simulink model "V5_2016_1"  (R2016a)
settings: Solver=VariableStepAuto  SolverMode=SingleTasking  StartTime=0.0  StopTime=60  RelTol=1e-3
values from neighbouring files (symbols this model uses):
  Ar = pi * (Lr^2) / 4    (= 0.0126676869774)    [Barrowman_Equations.m]    (also in barrowaman.mat)
  CD_data = CD{:, 2}    [Barrowman_Equations.m]    (also in barrowaman.mat = [0.48 0.48 0.47 0.46 0.45 0.44 0.43 0.42 0.42 0.41 0.4 0.4 .)
  CD_input = CD{:, 1}    [Barrowman_Equations.m]    (also in barrowaman.mat = [0.01 0.02 0.03 0.04 0.05 0.06 0.07 0.08 0.09 0.1 0.11 0.12 )
  Cnalfa = (Cnab + Cnalfat + Cntail)    [Barrowman_Equations.m]    (also in barrowaman.mat = 8.08141723415)
  Cndomega = (N * Cnalfa0 * Lr * (c1 + c2 + c3))/(Ar * span * (Lr))    [Barrowman_Equations.m]
  Cnfdelta = N * Cnalfa1 * Y / span    [Barrowman_Equations.m]    (also in barrowaman.mat = 4.20666666667)
  delta = pi/60    (= 0.0523598775598)    [Barrowman_Equations.m]    (also in barrowaman.mat = 0.00872664625997)
  F = readtable('Data/Comercial/Pro75M3100_saida_do_trilho.csv')    [Barrowman_Equations.m]
  F_data = F{:, 2}    [Barrowman_Equations.m]    (also in barrowaman.mat = [3391.768 3665.504 3532.913 3357.551 3199.297 3139.417 2412.)
  F_input = F{:, 1}    [Barrowman_Equations.m]    (also in barrowaman.mat = [0.02 0.057 0.148 0.496 0.817 0.936 1.173 1.501 1.717 1.78 1)
  mdescarregado = 15.576    [Barrowman_Equations.m]    (also in barrowaman.mat)
  MDot_data = MDot{:, 2}    [Barrowman_Equations.m]    (also in barrowaman.mat = [-1.96086837808 -2.11912220509 -2.04246793537 -1.9410866497 )
  MDot_input = MDot{:, 1}    [Barrowman_Equations.m]    (also in barrowaman.mat = [0.02 0.057 0.148 0.496 0.817 0.936 1.173 1.501 1.717 1.78 1)
  r = rt/r2    (= 1.45977011494)    [Barrowman_Equations.m]    (also in barrowaman.mat)
  x_cg = -1.278    [Barrowman_Equations.m]    (also in barrowaman.mat)
  x_ref = (XB * Cnab + XTB * Cnalfat + Xtail * Cntail) / Cnalfa    [Barrowman_Equations.m]    (also in barrowaman.mat = -1.69759908608)
undefined symbols (not defined in the file or in its folder): Light, MIL
libraries: aerolibasang x3, aerolibwind2 x3, aerolibatmos2 x1, aerolib6dof2 x1
settings Model: Creator=bruno  LastModifiedBy=patri
settings DataIOCC: ReturnWorkspaceOutputs=on
settings DebuggingCC: SFUnexpectedBacktrackingDiag=error  SFNoUnconditionalDefaultTransitionDiag=error
settings SFSimCC: SimUseLocalCustomCode=on
settings RTWCC: RTWUseLocalCustomCode=on
settings GRTTargetCC: TargetLangStandard=C99 (ISO)  GeneratePreprocessorConditionals=Use local settings
settings ConfigComp: CovMetricSettings=dwe  CovHtmlReporting=off  CovSaveCumulativeToWorkspaceVar=off  CovSaveSingleToWorkspaceVar=off  CovExternalEMLEnable=on

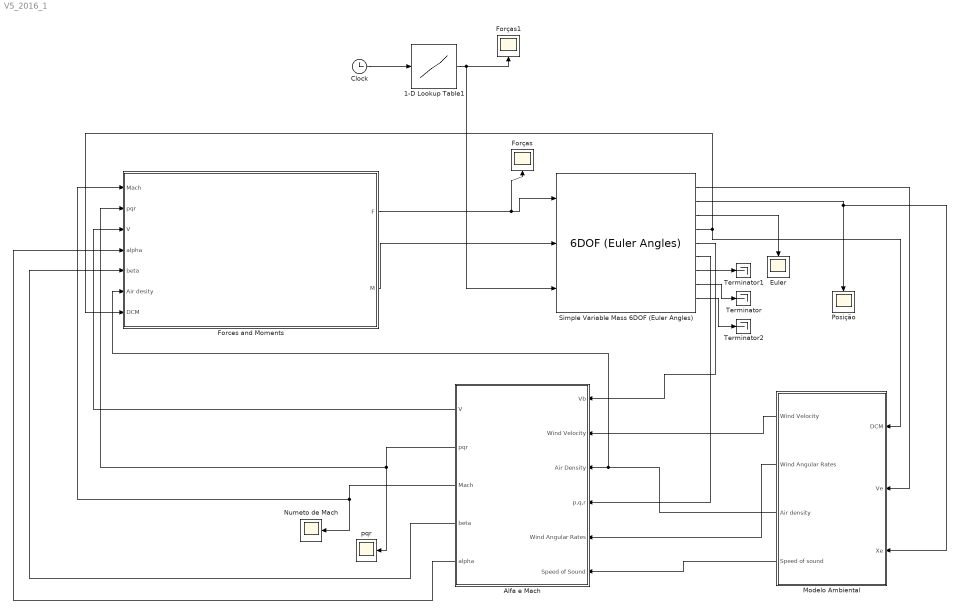
== system V5_2016_1 ==
  1-D Lookup Table1 : Lookup_n-D  NumberOfTableDimensions=1  BreakpointsForDimension1=MDot_input  Table=MDot_data  InternalRulePriority=Speed  RndMeth=Simplest  InputSameDT=on
  Alfa e Mach : Subsystem
  Clock : Clock
  Euler : Scope
  "Forces and Moments " : Subsystem
  Forças : Scope
  Forças1 : Scope
  Modelo Ambiental : Subsystem
  Numeto de Mach : Scope
  "Posição " : Scope
  Simple Variable Mass 6DOF (Euler Angles) : aerolib6dof2/6DOF (Euler Angles)  units=Metric (MKS)  mtype=Simple Variable  rep=Euler Angles  xme_0=[5 0 0]  Vm_0=[38 0 0]  eul_0=[0 -pi/2 0]  pm_0=[0 0 0]  mass_0=mcarregado  mass_e=mdescarregado  mass_f=mcarregado  inertia=eye(3)  inertia_e=MatrizDeInerciaDescarregado  inertia_f=MatrizDeInercia  k_quat=1.0  vre_flag=off
  Terminator : Terminator
  Terminator1 : Terminator
  Terminator2 : Terminator
  "pqr " : Scope
  wires:
  Simple Variable Mass 6DOF (Euler Angles)/4 -> Modelo Ambiental/1(DCM), "Forces and Moments "/7(DCM)
  Simple Variable Mass 6DOF (Euler Angles)/1 -> Modelo Ambiental/2(Ve)
  Simple Variable Mass 6DOF (Euler Angles)/2 -> "Posição "/1, Modelo Ambiental/3(Xe)
  Modelo Ambiental/3(Air density) -> "Forces and Moments "/6(Air desity), Alfa e Mach/3(Air Density)
  Modelo Ambiental/1(Wind Velocity) -> Alfa e Mach/2(Wind Velocity)
  Simple Variable Mass 6DOF (Euler Angles)/5 -> Alfa e Mach/1(Vb)
  Simple Variable Mass 6DOF (Euler Angles)/6 -> Alfa e Mach/4(p,q,r)
  Modelo Ambiental/4(Speed of sound) -> Alfa e Mach/6(Speed of Sound)
  Modelo Ambiental/2(Wind Angular Rates) -> Alfa e Mach/5(Wind Angular Rates)
  Alfa e Mach/3(Mach) -> Numeto de Mach/1, "Forces and Moments "/1(Mach)
  Alfa e Mach/2(pqr) -> "pqr "/1, "Forces and Moments "/2(pqr)
  Alfa e Mach/1(V) -> "Forces and Moments "/3("V ")
  Simple Variable Mass 6DOF (Euler Angles)/3 -> Euler/1
  Alfa e Mach/5("alpha ") -> "Forces and Moments "/4("alpha ")
  Alfa e Mach/4(beta) -> "Forces and Moments "/5(beta)
  "Forces and Moments "/1(F) -> Simple Variable Mass 6DOF (Euler Angles)/1, Forças/1
  Simple Variable Mass 6DOF (Euler Angles)/7 -> Terminator1/1
  Simple Variable Mass 6DOF (Euler Angles)/8 -> Terminator/1
  Clock/1 -> 1-D Lookup Table1/1
  1-D Lookup Table1/1 -> Simple Variable Mass 6DOF (Euler Angles)/3, Forças1/1
  Simple Variable Mass 6DOF (Euler Angles)/9 -> Terminator2/1
  "Forces and Moments "/2(M) -> Simple Variable Mass 6DOF (Euler Angles)/2

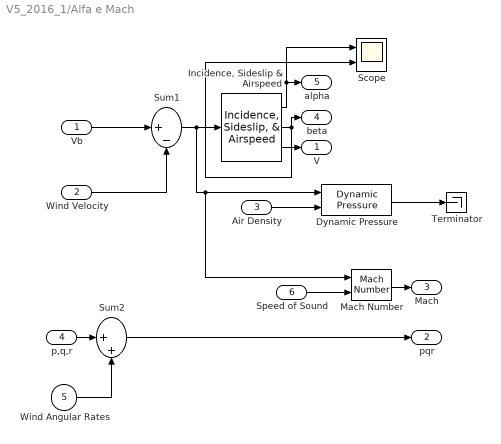
== system V5_2016_1/Alfa e Mach ==
  Vb : Inport
  Wind Velocity : Inport  Port=2
  Air Density : Inport  Port=3
  p,q,r : Inport  Port=4
  Wind Angular Rates : Inport  Port=5
  Speed of Sound : Inport  Port=6  Unit=m/s
  Dynamic Pressure : aerolibasang/Dynamic Pressure
  "Incidence, Sideslip & Airspeed" : aerolibasang/Incidence, Sideslip, & Airspeed
  Mach Number : aerolibasang/Mach Number
  Scope : Scope  NumInputPorts=2
  Sum1 : Sum  Inputs=|+-  SaturateOnIntegerOverflow=on  InputSameDT=on  OutDataTypeStr=Inherit: Same as first input
  Sum2 : Sum  Inputs=|++  SaturateOnIntegerOverflow=on  InputSameDT=on  OutDataTypeStr=Inherit: Same as first input
  Terminator : Terminator
  V : Outport
  pqr : Outport  Port=2
  Mach : Outport  Port=3
  beta : Outport  Port=4
  "alpha " : Outport  Port=5
  wires:
  Wind Velocity/1 -> Sum1/2
  Air Density/1 -> Dynamic Pressure/2
  Dynamic Pressure/1 -> Terminator/1
  "Incidence, Sideslip & Airspeed"/3 -> V/1
  p,q,r/1 -> Sum2/1
  Wind Angular Rates/1 -> Sum2/2
  Sum2/1 -> pqr/1
  Vb/1 -> Sum1/1
  Mach Number/1 -> Mach/1
  Sum1/1 -> Mach Number/1, Dynamic Pressure/1, "Incidence, Sideslip & Airspeed"/1
  Speed of Sound/1 -> Mach Number/2
  "Incidence, Sideslip & Airspeed"/2 -> beta/1, Scope/2
  "Incidence, Sideslip & Airspeed"/1 -> Scope/1, "alpha "/1

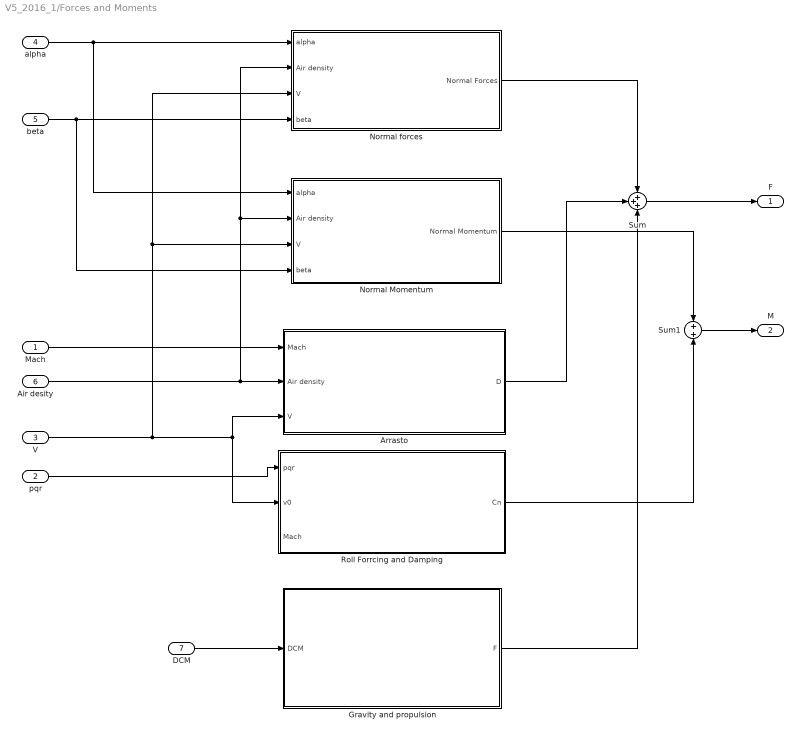
== system V5_2016_1/Forces and Moments  ==
  Mach : Inport
  pqr : Inport  Port=2
  "V " : Inport  Port=3
  "alpha " : Inport  Port=4
  beta : Inport  Port=5
  Air desity : Inport  Port=6
  DCM : Inport  Port=7
  Arrasto : Subsystem
  Gravity and propulsion : Subsystem
  Normal Momentum : Subsystem
  "Normal forces " : Subsystem
  Roll Forrcing and Damping : Subsystem
  Sum : Sum  Inputs=3
  Sum1 : Sum  Inputs=2
  F : Outport
  M : Outport  Port=2
  wires:
  Mach/1 -> Arrasto/1(Mach)
  pqr/1 -> Roll Forrcing and Damping/1(pqr)
  "V "/1 -> Normal Momentum/3(V), "Normal forces "/3("V "), Roll Forrcing and Damping/2("v0 "), Arrasto/3("V ")
  "alpha "/1 -> "Normal forces "/1("alpha "), Normal Momentum/1(alpha)
  Air desity/1 -> "Normal forces "/2(Air density), Normal Momentum/2(Air density), Arrasto/2(Air density)
  beta/1 -> Normal Momentum/4(beta), "Normal forces "/4(beta)
  Sum/1 -> F/1
  Gravity and propulsion/1(F) -> Sum/3
  DCM/1 -> Gravity and propulsion/1(DCM)
  Arrasto/1(D) -> Sum/2
  "Normal forces "/1(Normal Forces) -> Sum/1
  Roll Forrcing and Damping/1(Cn) -> Sum1/2
  Normal Momentum/1(Normal Momentum) -> Sum1/1
  Sum1/1 -> M/1

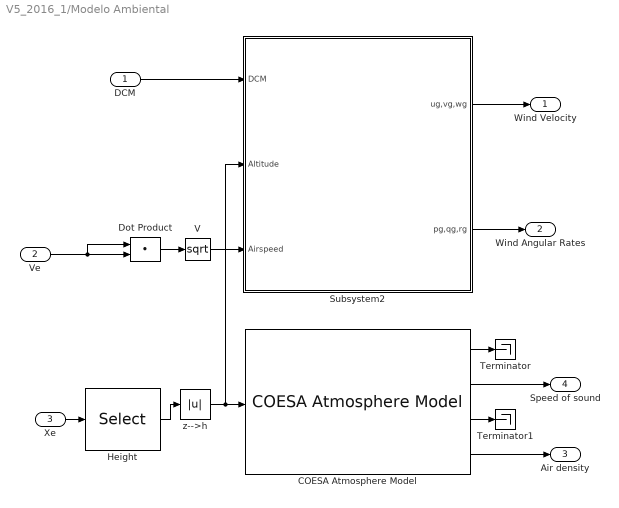
== system V5_2016_1/Modelo Ambiental ==
  DCM : Inport
  Ve : Inport  Port=2
  Xe : Inport  Port=3
  COESA Atmosphere Model : aerolibatmos2/COESA Atmosphere Model  units=Metric (MKS)  spec=1976 COESA-extended U.S. Standard Atmosphere  model=Profile  profile_var=High temperature  profile_percent=10%  profile_alt=5 km (16404 ft)  envelope_var=High temperature  envelope_percent=1%  action=None
  Dot Product : DotProduct  SaturateOnIntegerOverflow=on  OutDataTypeStr=Inherit: Inherit via internal rule
  Height : Selector  InputPortWidth=3  IndexOptions=Index vector (dialog)  Indices=[3]  OutputSizes=1
  Subsystem2 : Subsystem
  Terminator : Terminator
  Terminator1 : Terminator
  V : Math  Operator=sqrt  SaturateOnIntegerOverflow=on
  z-->h : Abs  SaturateOnIntegerOverflow=on
  Wind Velocity : Outport
  Wind Angular Rates : Outport  Port=2
  Air density : Outport  Port=3
  Speed of sound : Outport  Port=4
  wires:
  z-->h/1 -> Subsystem2/2(Altitude), COESA Atmosphere Model/1
  Subsystem2/1(ug,vg,wg) -> Wind Velocity/1
  Subsystem2/2(pg,qg,rg) -> Wind Angular Rates/1
  DCM/1 -> Subsystem2/1(DCM)
  Ve/1 -> Dot Product/1, Dot Product/2
  Dot Product/1 -> V/1
  V/1 -> Subsystem2/3(Airspeed)
  COESA Atmosphere Model/2 -> Speed of sound/1
  COESA Atmosphere Model/3 -> Terminator1/1
  COESA Atmosphere Model/1 -> Terminator/1
  COESA Atmosphere Model/4 -> Air density/1
  Height/1 -> z-->h/1
  Xe/1 -> Height/1

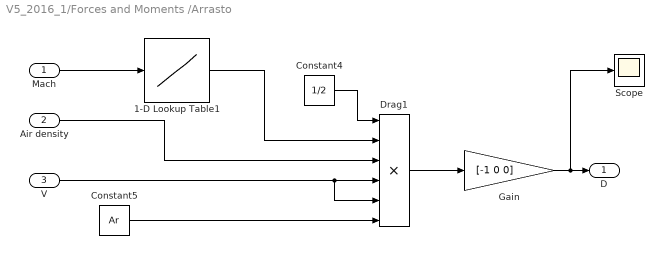
== system V5_2016_1/Forces and Moments /Arrasto ==
  Mach : Inport
  Air density : Inport  Port=2
  "V " : Inport  Port=3
  1-D Lookup Table1 : Lookup_n-D  NumberOfTableDimensions=1  BreakpointsForDimension1=CD_input  Table=CD_data  InternalRulePriority=Speed  RndMeth=Simplest  InputSameDT=on
  Constant4 : Constant  Value=1/2
  Constant5 : Constant  Value=Ar
  Drag1 : Product  Inputs=6
  Gain : Gain  Gain=[-1 0 0]
  Scope : Scope
  D : Outport
  wires:
  Mach/1 -> 1-D Lookup Table1/1
  Gain/1 -> Scope/1, D/1
  Drag1/1 -> Gain/1
  Constant4/1 -> Drag1/1
  1-D Lookup Table1/1 -> Drag1/2
  "V "/1 -> Drag1/5, Drag1/4
  Constant5/1 -> Drag1/6
  Air density/1 -> Drag1/3

== system V5_2016_1/Forces and Moments /Gravity and propulsion ==
  DCM : Inport
  "Gravidade " : Subsystem
  "Propulsão " : Subsystem
  Scope : Scope
  Scope1 : Scope
  Sum : Sum  Inputs=|++
  F : Outport
  wires:
  Sum/1 -> F/1
  "Propulsão "/1(F motor) -> Scope1/1, Sum/1
  DCM/1 -> "Gravidade "/1(DCM)
  "Gravidade "/1("F_gravidade ") -> Sum/2, Scope/1

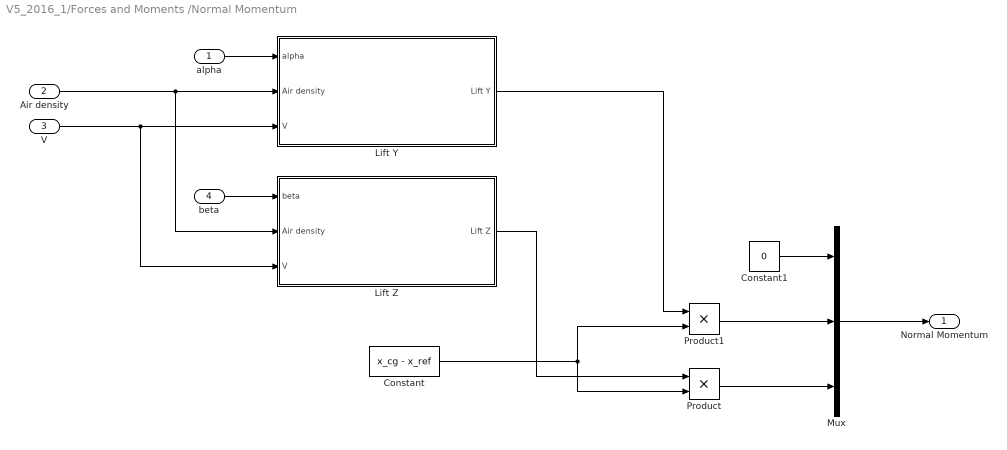
== system V5_2016_1/Forces and Moments /Normal Momentum ==
  alpha : Inport
  Air density : Inport  Port=2
  V : Inport  Port=3
  beta : Inport  Port=4
  Constant : Constant  Value=x_cg - x_ref
  Constant1 : Constant  Value=0
  Lift Y : Subsystem
  Lift Z : Subsystem
  Mux : Mux  Inputs=3
  Product : Product
  Product1 : Product
  Normal Momentum : Outport
  wires:
  Constant/1 -> Product/2, Product1/2
  Lift Z/1(Lift Z) -> Product/1
  V/1 -> Lift Y/3("V "), Lift Z/3("V ")
  Air density/1 -> Lift Y/2(Air density), Lift Z/2(Air density)
  Lift Y/1(Lift Y) -> Product1/1
  Mux/1 -> Normal Momentum/1
  Constant1/1 -> Mux/1
  alpha/1 -> Lift Y/1("alpha ")
  beta/1 -> Lift Z/1("beta ")
  Product1/1 -> Mux/2
  Product/1 -> Mux/3

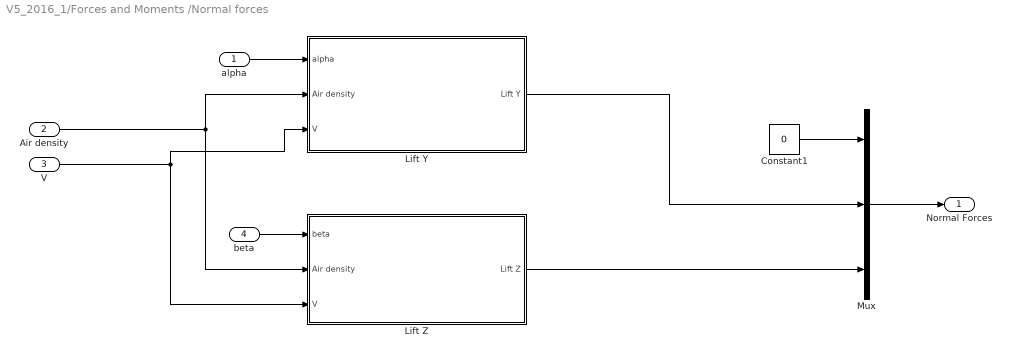
== system V5_2016_1/Forces and Moments /Normal forces  ==
  "alpha " : Inport
  Air density : Inport  Port=2
  "V " : Inport  Port=3
  beta : Inport  Port=4
  Constant1 : Constant  Value=0
  Lift Y : Subsystem
  Lift Z : Subsystem
  Mux : Mux  Inputs=3
  Normal Forces : Outport
  wires:
  Constant1/1 -> Mux/1
  Mux/1 -> Normal Forces/1
  "alpha "/1 -> Lift Y/1("alpha ")
  Air density/1 -> Lift Y/2(Air density), Lift Z/2(Air density)
  "V "/1 -> Lift Y/3("V "), Lift Z/3("V ")
  Lift Y/1(Lift Y) -> Mux/2
  beta/1 -> Lift Z/1("beta ")
  Lift Z/1(Lift Z) -> Mux/3

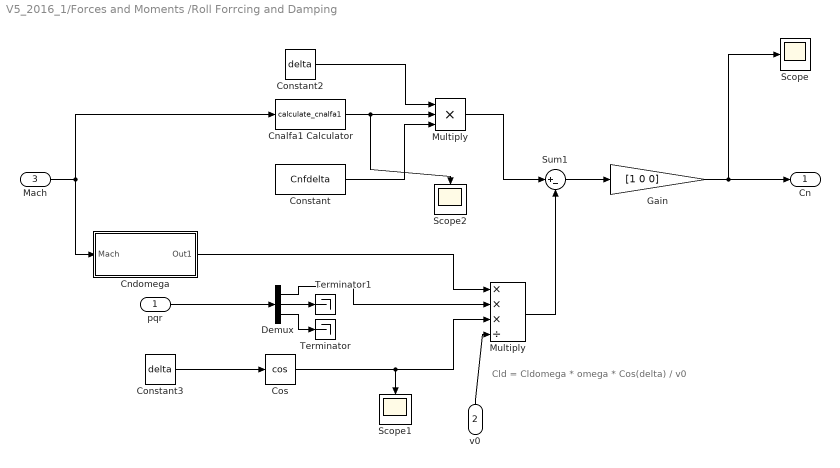
== system V5_2016_1/Forces and Moments /Roll Forrcing and Damping ==
  note: Cld = Cldomega * omega * Cos(delta) / v0
  pqr : Inport
  "v0 " : Inport  Port=2
  "Mach " : Inport  Port=3
  "Cnalfa1 Calculator " : MATLABFcn  MATLABFcn=calculate_cnalfa1
  "Cndomega " : Subsystem
  Constant : Constant  Value=Cnfdelta
  Constant2 : Constant  Value=delta
  Constant3 : Constant  Value=delta
  Cos : Trigonometry  Operator=cos
  Demux : Demux  Outputs=3
  Gain : Gain  Gain=[1 0 0]
  "Multiply " : Product  Inputs=***
  "Multiply " : Product  Inputs=***/
  Scope : Scope
  Scope1 : Scope
  Scope2 : Scope
  Sum1 : Sum  Inputs=|+-
  Terminator : Terminator
  Terminator1 : Terminator
  Cn : Outport
  wires:
  Constant2/1 -> "Multiply "/1
  "v0 "/1 -> "Multiply "/4
  "Multiply "/1 -> Sum1/1
  pqr/1 -> Demux/1
  Sum1/1 -> Gain/1
  Constant/1 -> "Multiply "/3
  Demux/2 -> Terminator1/1
  "Multiply "/1 -> Sum1/2
  Gain/1 -> Scope/1, Cn/1
  Constant3/1 -> Cos/1
  Cos/1 -> Scope1/1, "Multiply "/3
  Demux/3 -> Terminator/1
  Demux/1 -> "Multiply "/2
  "Mach "/1 -> "Cnalfa1 Calculator "/1, "Cndomega "/1("Mach ")
  "Cndomega "/1(Out1) -> "Multiply "/1
  "Cnalfa1 Calculator "/1 -> Scope2/1, "Multiply "/2

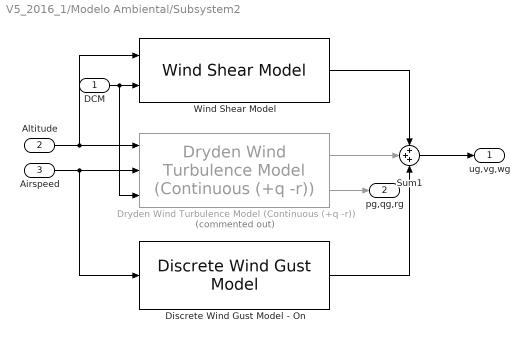
== system V5_2016_1/Modelo Ambiental/Subsystem2 ==
  DCM : Inport
  Altitude : Inport  Port=2
  Airspeed : Inport  Port=3
  Discrete Wind Gust Model - On : aerolibwind2/Discrete Wind Gust Model  units=Metric (MKS)  Gx=on  Gy=on  Gz=on  t_0=20  d_m=[120 120 80]  v_m=[3.5 3.0 3.0]
  Dryden Wind Turbulence Model (Continuous (+q -r)) : aerolibwind2/Dryden Wind Turbulence Model  (Continuous (+q -r))  Commented=on  units=Metric (MKS)  spec=MIL-F-8785C  model=Continuous Dryden (+q -r)  W20=5  Wdeg=0  TurbProb=10^-2 - Light  L_high=533.4  Wingspan=4  ts=0.1  Seed=[23341 23342 23343 23344]  T_on=on
  Sum1 : Sum  Inputs=+++  SaturateOnIntegerOverflow=on  InputSameDT=on  OutDataTypeStr=Inherit: Same as first input
  Wind Shear Model : aerolibwind2/Wind Shear Model  units=Metric (MKS)  phase=Category C - Terminal Flight Phase  W_20=1  Wdeg=0
  ug,vg,wg : Outport
  pg,qg,rg : Outport  Port=2
  wires:
  Dryden Wind Turbulence Model (Continuous (+q -r))/2 -> pg,qg,rg/1
  Wind Shear Model/1 -> Sum1/1
  Dryden Wind Turbulence Model (Continuous (+q -r))/1 -> Sum1/2
  Discrete Wind Gust Model - On/1 -> Sum1/3
  DCM/1 -> Dryden Wind Turbulence Model (Continuous (+q -r))/3, Wind Shear Model/2
  Airspeed/1 -> Dryden Wind Turbulence Model (Continuous (+q -r))/2, Discrete Wind Gust Model - On/1
  Sum1/1 -> ug,vg,wg/1
  Altitude/1 -> Dryden Wind Turbulence Model (Continuous (+q -r))/1, Wind Shear Model/1

== system V5_2016_1/Forces and Moments /Gravity and propulsion/Gravidade  ==
  DCM : Inport
  Constant1 : Constant  Value=9.81*mdescarregado
  Gain3 : Gain  Gain=[0 0 -1]
  Inertial to Body : Product  Multiplication=Matrix(*)  SaturateOnIntegerOverflow=on  InputSameDT=on  OutDataTypeStr=Inherit: Same as first input
  "F_gravidade " : Outport
  wires:
  Inertial to Body/1 -> "F_gravidade "/1
  DCM/1 -> Inertial to Body/1
  Gain3/1 -> Inertial to Body/2
  Constant1/1 -> Gain3/1

== system V5_2016_1/Forces and Moments /Gravity and propulsion/Propulsão  ==
  1-D Lookup Table : Lookup_n-D  NumberOfTableDimensions=1  BreakpointsForDimension1=F_input  Table=F_data  InternalRulePriority=Speed  RndMeth=Simplest  InputSameDT=on
  Clock1 : Clock
  Gain : Gain  Gain=[1 0 0]
  F motor : Outport
  wires:
  Gain/1 -> F motor/1
  Clock1/1 -> 1-D Lookup Table/1
  1-D Lookup Table/1 -> Gain/1

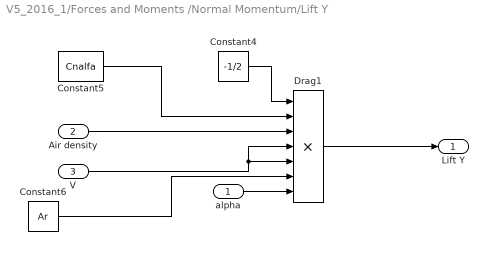
== system V5_2016_1/Forces and Moments /Normal Momentum/Lift Y ==
  "alpha " : Inport
  Air density : Inport  Port=2
  "V " : Inport  Port=3
  Constant4 : Constant  Value=-1/2
  Constant5 : Constant  Value=Cnalfa
  Constant6 : Constant  Value=Ar
  Drag1 : Product  Inputs=7
  Lift Y : Outport
  wires:
  "V "/1 -> Drag1/4, Drag1/5
  Constant6/1 -> Drag1/6
  Air density/1 -> Drag1/3
  "alpha "/1 -> Drag1/7
  Constant4/1 -> Drag1/1
  Constant5/1 -> Drag1/2
  Drag1/1 -> Lift Y/1

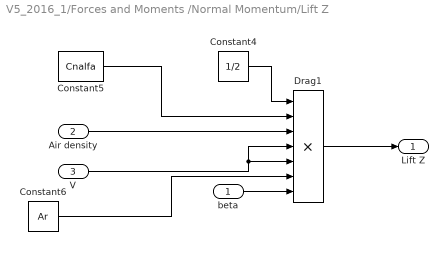
== system V5_2016_1/Forces and Moments /Normal Momentum/Lift Z ==
  "beta " : Inport
  Air density : Inport  Port=2
  "V " : Inport  Port=3
  Constant4 : Constant  Value=1/2
  Constant5 : Constant  Value=Cnalfa
  Constant6 : Constant  Value=Ar
  Drag1 : Product  Inputs=7
  Lift Z : Outport
  wires:
  "V "/1 -> Drag1/4, Drag1/5
  Constant6/1 -> Drag1/6
  Air density/1 -> Drag1/3
  "beta "/1 -> Drag1/7
  Constant4/1 -> Drag1/1
  Constant5/1 -> Drag1/2
  Drag1/1 -> Lift Z/1

== system V5_2016_1/Forces and Moments /Normal forces /Lift Y ==
  "alpha " : Inport
  Air density : Inport  Port=2
  "V " : Inport  Port=3
  Constant4 : Constant  Value=1/2
  Constant5 : Constant  Value=Cnalfa
  Constant6 : Constant  Value=Ar
  Drag1 : Product  Inputs=7
  Lift Y : Outport
  wires:
  "V "/1 -> Drag1/4, Drag1/5
  Constant6/1 -> Drag1/6
  Air density/1 -> Drag1/3
  "alpha "/1 -> Drag1/7
  Constant4/1 -> Drag1/1
  Constant5/1 -> Drag1/2
  Drag1/1 -> Lift Y/1

== system V5_2016_1/Forces and Moments /Normal forces /Lift Z ==
  "beta " : Inport
  Air density : Inport  Port=2
  "V " : Inport  Port=3
  Constant4 : Constant  Value=1/2
  Constant5 : Constant  Value=Cnalfa
  Constant6 : Constant  Value=Ar
  Drag1 : Product  Inputs=7
  Lift Z : Outport
  wires:
  "V "/1 -> Drag1/4, Drag1/5
  Constant6/1 -> Drag1/6
  Air density/1 -> Drag1/3
  "beta "/1 -> Drag1/7
  Constant4/1 -> Drag1/1
  Constant5/1 -> Drag1/2
  Drag1/1 -> Lift Z/1

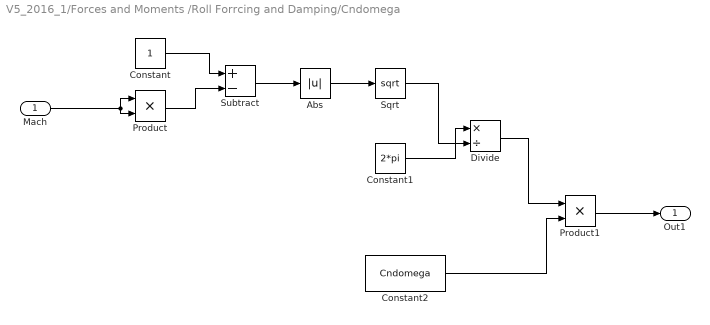
== system V5_2016_1/Forces and Moments /Roll Forrcing and Damping/Cndomega  ==
  "Mach " : Inport
  Abs : Abs
  Constant : Constant
  Constant1 : Constant  Value=2*pi
  Constant2 : Constant  Value=Cndomega
  Divide : Product  Inputs=*/
  Product : Product
  Product1 : Product
  Sqrt : Sqrt  SaturateOnIntegerOverflow=on
  Subtract : Sum  Inputs=+-
  Out1 : Outport
  wires:
  "Mach "/1 -> Product/1, Product/2
  Product/1 -> Subtract/2
  Constant/1 -> Subtract/1
  Subtract/1 -> Abs/1
  Abs/1 -> Sqrt/1
  Sqrt/1 -> Divide/2
  Constant1/1 -> Divide/1
  Divide/1 -> Product1/1
  Constant2/1 -> Product1/2
  Product1/1 -> Out1/1
